simulink model "psbdiode"  (Simulink 6.0)
settings: Solver=ode23tb  SolverMode=SingleTasking  StartTime=0.0  StopTime=0.06  FixedStep=100e-6  RelTol=1e-3  AbsTol=1e-2
libraries: powerlib2 x7
settings Model: Creator=patrice  LastModifiedBy=batserve  ExtModeTrigMode=oneshot  ExtModeArmWhenConnect=off  ExtModeAutoUpdateStatusClock=off
settings DataIOCC: LimitDataPoints=off  SaveOutput=off  SaveTime=off  TimeSaveName=t  SignalLoggingName=sigsOut
settings OptimizationCC: BlockReduction=off  BooleanDataType=off
settings DebuggingCC: SolverPrmCheckMsg=none
settings HardwareCC: TargetUnknown=on
settings RTWCC: TemplateMakefile=grt_unix.tmf

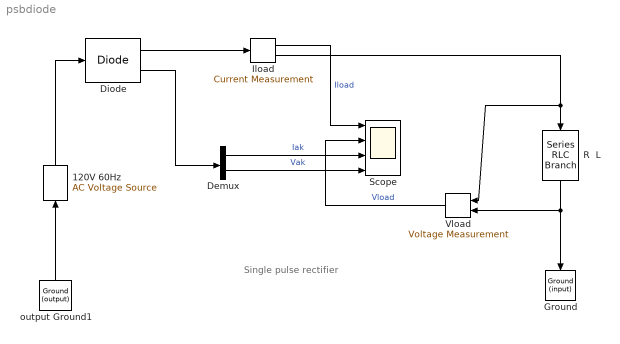
== system psbdiode ==
  note: Single pulse rectifier
  120V 60Hz : powerlib2/Electrical Sources/AC Voltage Source  Tag=PoWeRsYsTeMbLoCk  Orientation=up  A=120  P=0  F=60  stime=0  mesure=None  PSBOutputType=1
  Demux : Demux  Outputs=2
  Diode : powerlib2/Power Electronics/Diode  Tag=PoWeRsYsTeMbLoCk  Ron=0.001  Lon=1e-6  Vf=0.8  IC=0  Rs=20  Cs=4e-6  PSBOutputType=10
  Ground : powerlib2/Connectors/Ground (input)  Tag=PoWeRsYsTeMbLoCk  Orientation=down
  Iload : powerlib2/Measurements/Current Measurement  Tag=PoWeRsYsTeMmEaSuReMeNt  PhasorSimulation=off  OutputType=Magnitude  PSBOutputType=01  PSBequivalent=0
  R  L : powerlib2/Elements/Series RLC Branch  Tag=PoWeRsYsTeMbLoCk  Orientation=down  a=1  b=1e-03  c=inf  mesure=None  PSBOutputType=1
  Scope : Scope  NumInputPorts=4
      settings: TimeRange=0.06  YMin=-200~-200~0~-200  YMax=200~200~200~200  DataFormat=Array
  Vload : powerlib2/Measurements/Voltage Measurement  Tag=PoWeRsYsTeMmEaSuReMeNt  Orientation=left  PhasorSimulation=off  OutputType=Magnitude  PSBOutputType=0  PSBequivalent=0
  output Ground1 : powerlib2/Connectors/Ground (output)  Tag=PoWeRsYsTeMbLoCk  Orientation=up  PSBOutputType=1
  wires:
  Iload/2 -> R  L/1, Vload/1
  R  L/1 -> Ground/1, Vload/2
  Diode/1 -> Iload/1
  Diode/2 -> Demux/1
  output Ground1/1 -> 120V 60Hz/1
  120V 60Hz/1 -> Diode/1
  Iload/1 -> Scope/1  "Iload"
  Vload/1 -> Scope/2  "Vload"
  Demux/1 -> Scope/3  "Iak"
  Demux/2 -> Scope/4  "Vak"
